simulink model "zynq_learn_axistream"  (R2025b)
settings: Solver=FixedStepDiscrete  StartTime=0.0  StopTime=0.001  FixedStep=2e-08  RelTol=1e-3
libraries: simulink x1
settings Model: DataTypeOverride=Off  Creator=kimsteph  LastModifiedBy=kimsteph
settings OptimizationCC: BlockReduction=off  ConditionallyExecuteInputs=off  DefaultParameterBehavior=Inlined  InheritOutputTypeSmallerThanSingle=on
settings DebuggingCC: ArtificialAlgebraicLoopMsg=error  SingleTaskRateTransMsg=error
settings HardwareCC: ProdBitPerPointer=32.0  ProdBitPerSizeT=32.0  ProdBitPerPtrDiffT=32.0  ProdLargestAtomicFloat=None  ProdIntDivRoundTo=Undefined  ProdEndianess=Unspecified  ProdWordSize=32.0  ProdHWDeviceType=ASIC/FPGA->ASIC/FPGA  TargetBitPerPointer=64.0  TargetBitPerSizeT=64.0  TargetBitPerPtrDiffT=64.0  TargetLongLongMode=on  TargetIntDivRoundTo=Zero  TargetEndianess=LittleEndian  TargetWordSize=64.0  TargetHWDeviceType=Custom Processor->MATLAB Host Computer  ProdEqTarget=off

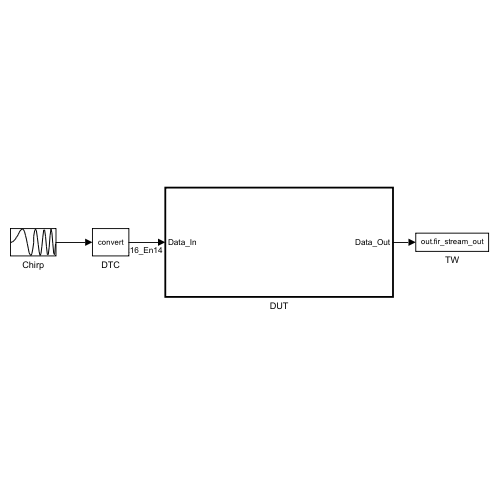
[thumbnail: Simulink's stored preview of the top-level diagram]
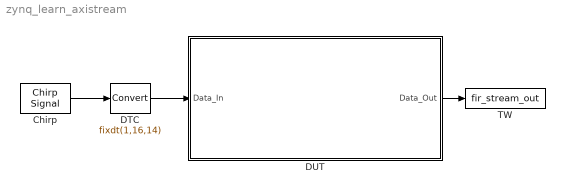
== system zynq_learn_axistream ==
  Chirp : simulink/Sources/Chirp Signal  f1=100  T=0.001  f2=5000
  DTC : DataTypeConversion  OutDataTypeStr=fixdt(1,16,14)  SaturateOnIntegerOverflow=off  RndMeth=Floor
  DUT : Subsystem  TreatAsAtomicUnit=on
  TW : ToWorkspace  VariableName=fir_stream_out  SaveFormat=Timeseries  SampleTime=-1
  wires:
  Chirp/1 -> DTC/1
  DTC/1 -> DUT/1(Data_In)
  DUT/1(Data_Out) -> TW/1

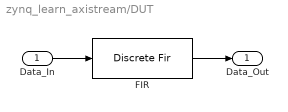
== system zynq_learn_axistream/DUT ==
  Data_In : Inport  OutDataTypeStr=fixdt(1,16,14)
  FIR : DiscreteFir  Coefficients=[0.02802 0.09763 0.166 0.2083 0.2083 0.166 0.09763 0.02802]  SampleTime=2e-08  CoefDataTypeStr=fixdt(1,16,14)  ProductDataTypeStr=fixdt(1,32,28)  AccumDataTypeStr=fixdt(1,32,28)  OutDataTypeStr=fixdt(1,16,14)
  Data_Out : Outport
  wires:
  Data_In/1 -> FIR/1
  FIR/1 -> Data_Out/1
